simulink model "Nmpc_pathctl_casadi"  (R2022b)
settings: Solver=FixedStepAuto  StartTime=0.0  StopTime=25  FixedStep=.001  MaxStep=0.01  RelTol=1e-3
values from neighbouring files (symbols this model uses):
  xuanze = Input(15)    [NMPC_casadi_yhn.m]    (also in plotfig.m = 0)
libraries: Solver_SF x1
(part 1 of 11)
settings Model: SimulationMode=accelerator  Creator=Murad  LastModifiedBy=gfr_love_myf
settings SolverCC: AlgebraicLoopSolver=LineSearch
settings OptimizationCC: EfficientMapNaN2IntZero=off
settings DebuggingCC: UnconnectedInputMsg=warning  UnconnectedOutputMsg=warning  UnconnectedLineMsg=warning  SFMachineParentedDataDiag=warning
settings HardwareCC: TargetBitPerPointer=64  TargetBitPerSizeT=64  TargetBitPerPtrDiffT=64  TargetLongLongMode=on  TargetIntDivRoundTo=Zero  TargetEndianess=LittleEndian  TargetWordSize=64  TargetHWDeviceType=MATLAB Host  ProdEqTarget=off
settings ModelReferenceCC: EnableRefExpFcnMdlSchedulingChecks=on
settings SFSimCC: CustomCodeUndefinedFunction=UseInterfaceOnly
settings CodeAppCC: MaxIdLength=128
settings GRTTargetCC: TargetLangStandard=C89/C90 (ANSI)  CombineOutputUpdateFcns=off  GRTInterface=on

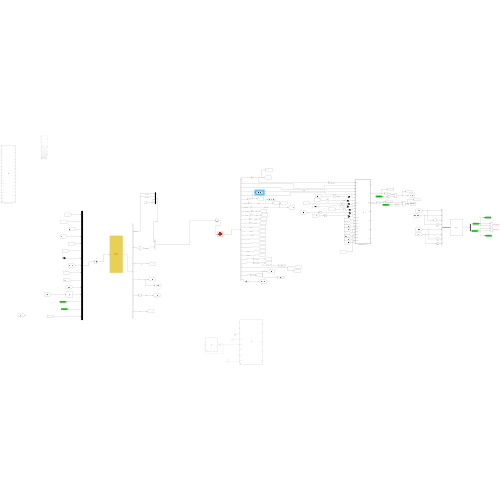
[thumbnail: Simulink's stored preview of the top-level diagram]
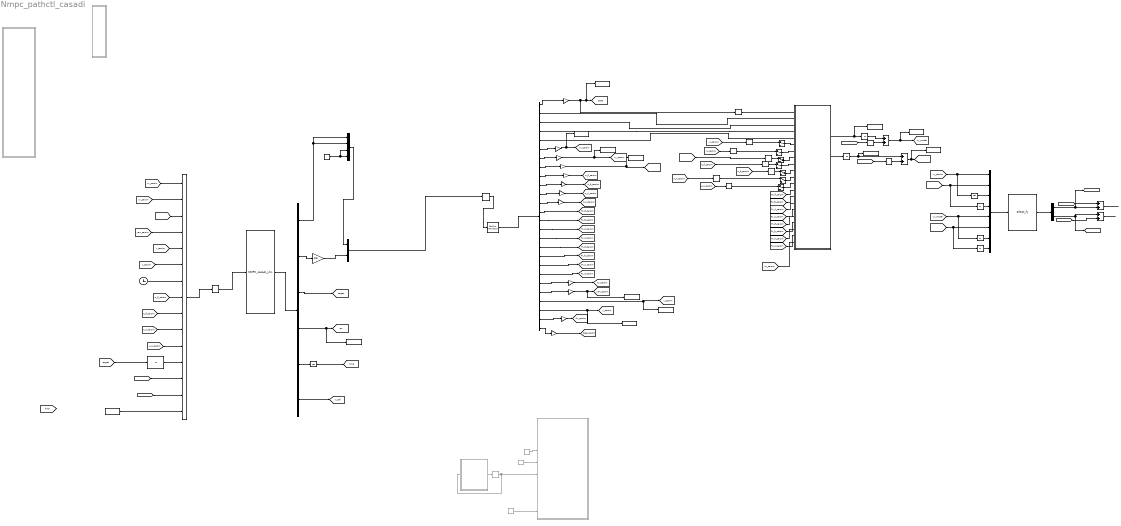
== system Nmpc_pathctl_casadi ==
  Add{1..4} (4 alike) : Sum
  Burckhardt轮胎侧向力_低附 : MATLAB Function  TreatAsAtomicUnit=on
  Burckhardt轮胎侧向力_低附1 : MATLAB Function  Commented=on  TreatAsAtomicUnit=on
  Bus Creator : BusCreator  Inputs=8
  CarSim S-Function : Solver_SF/CarSim S-Function  Priority=1  SIMFILE=simfile.sim  Run_RTs=off  vs_state_ind=Run  StopMode_ind=Vehicle Model
  Clock : Clock
  Constant : Constant  Value=0
  Constant1 : Constant  Commented=on  Value=10
  Constant2 : Constant  Commented=on  Value=10
  Constant3 : Constant  Commented=on  Value=10
  Constant4 : Constant  Value=xuanze
  Delay : Delay  Commented=on  DelayLength=1  InitialCondition=10
  Delay1 : Delay  DelayLength=1  InitialCondition=0
  Delay10 : Delay  DelayLength=15  InitialCondition=0
  Delay{2..5} (4 alike) : Delay  DelayLength=15  InitialCondition=8
  Delay6 : Delay  DelayLength=1  InitialCondition=10
  Delay7 : Delay  DelayLength=1  InitialCondition=0
  Delay8 : Delay  DelayLength=1  InitialCondition=0
  Delay9 : Delay  DelayLength=15  InitialCondition=0
  Demux : Demux  Outputs=2
  Demux1 : Demux  Outputs=6
  Demux2 : Demux  Outputs=26
  Gain : Gain  Gain=1/3.6
  Gain1 : Gain  Gain=1/3.6
  Gain10 : Gain  Gain=9.8
  Gain11 : Gain  Gain=400
  Gain{2,7,9,12} (4 alike) : Gain  Gain=pi/180
  Gain{3..6} (4 alike) : Gain  Gain=pi/30*0.3018
  Gain8 : Gain  Gain=9.8
  Interpreted MATLAB Function : MATLABFcn  MATLABFcn=NMPC_casadi_yhn  OutputDimensions=6  Output1D=off
  MATLAB Function1 : MATLAB Function  Commented=on  TreatAsAtomicUnit=on
  MATLAB Function2 : MATLAB Function  Commented=on  TreatAsAtomicUnit=on
  Manual Switch{,1..6} (7 alike) : ManualSwitch
  Mux : Mux  Inputs=2
  Mux1 : Mux  Inputs=15
  Mux2 : Mux
  Rate Transition1 : RateTransition  OutPortSampleTime=0.001
  Rate Transition2 : RateTransition  OutPortSampleTime=0.02
  S-Function1 : S-Function  FunctionName=adapt_fy  SFunctionDeploymentMode=off  EnableBusSupport=off
  To Workspace : ToWorkspace  VariableName=y_carsim  SaveFormat=Timeseries  SampleTime=-1
  To Workspace1 : ToWorkspace  VariableName=x_carsim  SaveFormat=Timeseries  SampleTime=-1
  To Workspace10 : ToWorkspace  VariableName=vy_data  SaveFormat=Timeseries  SampleTime=-1
  To Workspace11 : ToWorkspace  VariableName=vx_carsim  SaveFormat=Timeseries  SampleTime=-1
  To Workspace2 : ToWorkspace  VariableName=err  SaveFormat=Timeseries  SampleTime=-1
  To Workspace3 : ToWorkspace  VariableName=yaw  SaveFormat=Timeseries  SampleTime=-1
  To Workspace4 : ToWorkspace  VariableName=delta  SaveFormat=Timeseries  SampleTime=-1
  To Workspace5 : ToWorkspace  VariableName=vy_com  SaveFormat=Timeseries  SampleTime=-1
  To Workspace6 : ToWorkspace  VariableName=gamma_com  SaveFormat=Timeseries  SampleTime=-1
  To Workspace7 : ToWorkspace  VariableName=gamma_model  SaveFormat=Timeseries  SampleTime=-1
  To Workspace8 : ToWorkspace  VariableName=vy_model  SaveFormat=Timeseries  SampleTime=-1
  To Workspace9 : ToWorkspace  VariableName=gamma_data  SaveFormat=Timeseries  SampleTime=-1
  Unit Delay{1..6,12} (7 alike) : UnitDelay  SampleTime=-1  HasFrameUpgradeWarning=on
  Unit Delay11 : UnitDelay  InitialCondition=1  SampleTime=-1  HasFrameUpgradeWarning=on
  刘胜涛师兄路径跟踪 : Subsystem  Commented=on
  tag scope: Ax_carsim=global, Ay_carsim=global, Fx_fl_carsim=global, Fx_fr_carsim=global, Fx_rl_carsim=global, Fx_rr_carsim=global, Fy_fl_carsim=global, Fy_fr_carsim=global, Fy_rl_carsim=global, Fy_rr_carsim=global, beta_carsim=global, delta=global, err=global, gamma_carsim=global, gamma_com=global, gamma_model=global, target=global, time=global, vx_carsim=global, vy_carsim=global, vy_com=global, vy_model=global, w_fl_carsim=global, w_fr_carsim=global, w_ref=global, w_rl_carsim=global, w_rr_carsim=global, x_carsim=global, y_carsim=global, yaw_carsim=global
  wires:
  Burckhardt轮胎侧向力_低附/3(gamma) -> Unit Delay5/1  "gamma_model"
  CarSim S-Function/1 -> Demux2/1
  Demux2/1 -> Gain7/1  "delta_carsim"
  Demux2/2 -> Burckhardt轮胎侧向力_低附/2(Tc_fl)  "Tc_fl_carsim"
  Demux2/3 -> Burckhardt轮胎侧向力_低附/3(Tc_fr)  "Tc_fr_carsim"
  Demux2/4 -> Burckhardt轮胎侧向力_低附/4(Tc_rl)  "Tc_rl_carsim"
  Demux2/5 -> Burckhardt轮胎侧向力_低附/5(Tc_rr)  "Tc_rr_carsim"
  Demux2/6 -> Gain/1  "vx_carsim"
  Demux2/7 -> Gain1/1  "vy_carsim"
  Demux2/8 -> Gain2/1  "gamma_carsim"
  Demux2/9 -> Gain3/1  "w_fl_carsim"
  Demux2/10 -> Gain4/1  "w_fr_carsim"
  Demux2/11 -> Gain5/1  "w_rl_carsim"
  Demux2/12 -> Gain6/1  "w_rr_carsim"
  Gain1/1 -> To Workspace10/1, [vy_carsim]  "vy_carsim"
  Gain2/1 -> To Workspace9/1, [gamma_carsim]  "gamma_carsim"
  Gain3/1 -> [w_fl_carsim]  "w_fl_carsim"
  Gain4/1 -> [w_fr_carsim]  "w_fr_carsim"
  Gain5/1 -> [w_rl_carsim]  "w_rl_carsim"
  Gain6/1 -> [w_rr_carsim]  "w_rr_carsim"
  [vx_carsim] -> Delay6/1
  Manual Switch/1 -> Burckhardt轮胎侧向力_低附/6("vx ")
  Manual Switch1/1 -> Burckhardt轮胎侧向力_低附/7("vy ")
  [vy_carsim] -> Delay7/1
  [gamma_carsim] -> Delay8/1
  Manual Switch2/1 -> Burckhardt轮胎侧向力_低附/8("gamma ")
  Manual Switch3/1 -> Burckhardt轮胎侧向力_低附/9(w_fl)
  Manual Switch4/1 -> Burckhardt轮胎侧向力_低附/10(w_fr)
  Manual Switch5/1 -> Burckhardt轮胎侧向力_低附/11(w_rl)
  Manual Switch6/1 -> Burckhardt轮胎侧向力_低附/12(w_rr)
  Demux2/13 -> [Fy_fl_carsim]  "Fyfl_carsim"
  Demux2/14 -> [Fy_fr_carsim]  "Fyfr_carsim"
  Demux2/15 -> [Fy_rl_carsim]  "Fyrl_carsim"
  Demux2/16 -> [Fy_rr_carsim]  "Fyrr_carsim"
  Demux2/20 -> [Fx_rr_carsim]  "Fxrr_carsim"
  Demux2/18 -> [Fx_fr_carsim]  "Fxfr_carsim"
  Demux2/19 -> [Fx_rl_carsim]  "Fxrl_carsim"
  Demux2/17 -> [Fx_fl_carsim]  "Fxfl_carsim"
  [Fy_fl_carsim] -> Burckhardt轮胎侧向力_低附/13(fyfl_carsim)
  [Fy_fr_carsim] -> Burckhardt轮胎侧向力_低附/14(fyfr_carsim)
  [Fy_rl_carsim] -> Burckhardt轮胎侧向力_低附/15(fyrl_carsim)
  [Fy_rr_carsim] -> Burckhardt轮胎侧向力_低附/16(fyrr_carsim)
  [Fx_fl_carsim] -> Burckhardt轮胎侧向力_低附/17(fxfl_carsim)
  [Fx_fr_carsim] -> Burckhardt轮胎侧向力_低附/18(fxfr_carsim)
  [Fx_rl_carsim] -> Burckhardt轮胎侧向力_低附/19(fxrl_carsim)
  [Fx_rr_carsim] -> Burckhardt轮胎侧向力_低附/20(fxrr_carsim)
  Gain7/1 -> To Workspace4/1, [delta], Delay1/1  "delta_carsim"
  Demux2/21 -> Gain8/1  "Ay_carsim"
  Gain8/1 -> [Ay_carsim]  "Ay_carsim"
  [vy_carsim] -> Bus Creator/1, Unit Delay1/1
  [gamma_carsim] -> Unit Delay2/1, Bus Creator/2
  Unit Delay1/1 -> Bus Creator/3
  Unit Delay2/1 -> Bus Creator/4
  [vy_model] -> Unit Delay3/1, Bus Creator/5
  [gamma_model] -> Unit Delay4/1, Bus Creator/6
  Unit Delay4/1 -> Bus Creator/8
  Unit Delay3/1 -> Bus Creator/7
  Bus Creator/1 -> S-Function1/1
  Add2/1 -> ?  "Vy_com"
  S-Function1/1 -> Demux/1
  [vy_model] -> Add2/1
  Demux/2 -> [gamma_com], Add3/1
  Add3/1 -> ?  "gamma_com"
  Demux/1 -> Add2/2, [vy_com]
  [gamma_model] -> Add3/2
  Burckhardt轮胎侧向力_低附/2(vy) -> To Workspace8/1, Unit Delay6/1  "vy_model"
  [vy_com] -> Delay9/1
  Demux2/22 -> Gain9/1
  Gain9/1 -> To Workspace3/1, [yaw_carsim]  "yaw_carsim"
  Demux2/23 -> [x_carsim], To Workspace1/1  "x_carsim"
  Demux2/24 -> [y_carsim], To Workspace/1  "y_carsim"
  Demux2/25 -> Gain10/1
  Gain10/1 -> [Ax_carsim]  "Ax_carsim"
  Delay6/1 -> Manual Switch/1  "w_fl_model"
  Delay7/1 -> Manual Switch1/1  "w_fl_model"
  Delay8/1 -> Manual Switch2/1  "w_fl_model"
  [gamma_com] -> Delay10/1
  Add1/1 -> To Workspace5/1, [vy_model]  "Vy_com"
  Add4/1 -> To Workspace6/1, [gamma_model]  "gamma_com"
  [Ax_carsim] -> Burckhardt轮胎侧向力_低附/21(ax_carsim)
  [w_fl_carsim] -> Delay2/1
  [w_fr_carsim] -> Delay3/1
  [w_rl_carsim] -> Delay4/1
  [w_rr_carsim] -> Delay5/1
  Delay2/1 -> Manual Switch3/1
  Delay3/1 -> Manual Switch4/1
  Delay4/1 -> Manual Switch5/1
  Delay5/1 -> Manual Switch6/1
  Delay1/1 -> Burckhardt轮胎侧向力_低附/1(delta)  "w_fl_model"
  Delay9/1 -> Add1/2
  Delay10/1 -> Add4/2
  Interpreted MATLAB Function/1 -> Demux1/1
  Demux1/1 -> Mux2/2, Mux2/1  "delta_carsim"
  Constant/1 -> Mux2/3, Mux2/4
  Mux2/1 -> Mux/1
  Rate Transition1/1 -> CarSim S-Function/1
  Demux1/2 -> Gain11/1  "ax"
  Gain11/1 -> Mux/2  "T_emergine"
  [vx_carsim] -> Mux1/1
  [vy_carsim] -> Mux1/2
  [gamma_carsim] -> Mux1/3
  [yaw_carsim] -> Mux1/4
  [x_carsim] -> Mux1/5
  [y_carsim] -> Mux1/6
  Mux1/1 -> Rate Transition2/1
  Rate Transition2/1 -> Interpreted MATLAB Function/1
  [w_fl_carsim] -> Mux1/8
  [w_fr_carsim] -> Mux1/9
  [w_rl_carsim] -> Mux1/10
  [w_rr_carsim] -> Mux1/11
  Unit Delay5/1 -> To Workspace7/1, Add4/1  "w_fr_model"
  Unit Delay6/1 -> Add1/1  "w_fr_model"
  Clock/1 -> Mux1/7  "t"
  Demux1/3 -> [target]  "taget"
  Mux/1 -> Rate Transition1/1
  Unit Delay11/1 -> Mux1/12
  [target] -> Unit Delay11/1
  Demux1/4 -> To Workspace2/1, [err]  "err"
  Constant1/1 -> MATLAB Function1/8(target)
  MATLAB Function2/1(y) -> Delay/1
  Delay/1 -> MATLAB Function2/1(u), MATLAB Function1/5(curvepos0)  "x"
  Constant2/1 -> MATLAB Function1/4(lamada)
  Constant3/1 -> MATLAB Function1/3(z)
  Demux1/5 -> Unit Delay12/1
  Unit Delay12/1 -> [time]  "time"
  Demux2/26 -> Gain12/1
  Gain12/1 -> [beta_carsim]  "beta_carsim"
  Demux1/6 -> [w_ref]  "w_ref"
  Constant4/1 -> Mux1/15
  [vy_com] -> Mux1/13
  [gamma_com] -> Mux1/14
  Gain/1 -> To Workspace11/1, [vx_carsim]  "err"

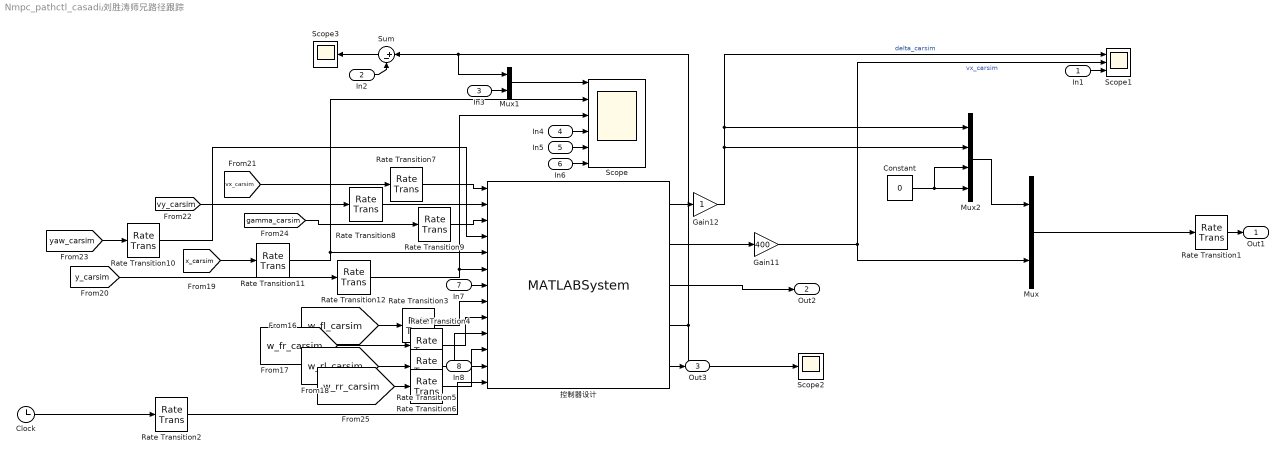
== system Nmpc_pathctl_casadi/刘胜涛师兄路径跟踪 ==
  In1 : Inport
  In2 : Inport  Port=2
  In3 : Inport  Port=3
  In4 : Inport  Port=4
  In5 : Inport  Port=5
  In6 : Inport  Port=6
  In7 : Inport  Port=7
  In8 : Inport  Port=8
  Clock : Clock
  Constant : Constant  Value=0
  Gain11 : Gain  Gain=400
  Gain12 : Gain
  Mux : Mux  Inputs=2
  Mux1 : Mux  Inputs=2
  Mux2 : Mux
  Rate Transition1 : RateTransition  OutPortSampleTime=0.001
  Rate Transition{2,7..11} (6 alike) : RateTransition  OutPortSampleTime=0.02
  Rate Transition{3..6,12} (5 alike) : RateTransition  OutPortSampleTime=0.1
  Scope : Scope  NumInputPorts=6
  Scope1 : Scope  NumInputPorts=3
  Scope2 : Scope
  Scope3 : Scope
  Sum : Sum  Inputs=|+-
  控制器设计 : MATLABSystem  System=NMPC_PCtl_casadi  SimulateUsing=Interpreted execution
      mask Type: NMPC_PCtl_casadi
      mask Display:
      | disp('NMPC_PCtl_casadi');
      | port_label('input',1,'xd_in');
      | port_label('input',2,'yd_in');
      | port_label('input',3,'yawd_in');
      | port_label('input',4,'yaw_in');
      | port_label('input',5,'x_in');
      | port_label('input',6,'y_in');
      | port_label('input',7,'w_fl');
      | port_label('input',8,'w_fr');
      | port_label('input',9,'w_rl');
      | port_label('input',10,'w_rr');
      | port_label('input',11,'vy_com');
      | port_label('input',12,'gamma_com');
      | port_label('input',13,'t');
      | port_label('output',1,'delta_out');
      | port_label('output',2,'acc_out');
      | port_label('output',3,'break_out');
      | port_label('output',4,'vref');
      | port_label('output',5,'target');
  Out1 : Outport
  Out2 : Outport  Port=2
  Out3 : Outport  Port=3
  wires:
  Mux/1 -> Rate Transition1/1
  In4/1 -> Scope/4
  Rate Transition1/1 -> Out1/1
  Mux2/1 -> Mux/1
  Gain12/1 -> Scope1/1, Mux2/1, Mux2/2  "delta_carsim"
  Rate Transition4/1 -> 控制器设计/9
  Clock/1 -> Rate Transition2/1
  Sum/1 -> Scope3/1
  控制器设计/1 -> Gain12/1
  Rate Transition12/1 -> 控制器设计/6, Scope/3
  [w_rl_carsim] -> Rate Transition5/1
  Mux1/1 -> Scope/1
  控制器设计/2 -> Gain11/1
  [gamma_carsim] -> Rate Transition9/1
  Gain11/1 -> Mux/2, Scope1/2  "vx_carsim"
  [yaw_carsim] -> Rate Transition10/1
  In1/1 -> Scope1/3
  控制器设计/4 -> Scope2/1, Mux1/1, Sum/1
  [vy_carsim] -> Rate Transition8/1
  Rate Transition9/1 -> 控制器设计/3
  Constant/1 -> Mux2/3, Mux2/4
  [x_carsim] -> Rate Transition11/1
  Rate Transition6/1 -> 控制器设计/11
  [w_fr_carsim] -> Rate Transition4/1
  控制器设计/3 -> Out2/1
  In8/1 -> 控制器设计/12
  [w_fl_carsim] -> Rate Transition3/1
  [y_carsim] -> Rate Transition12/1
  Rate Transition5/1 -> 控制器设计/10
  Rate Transition8/1 -> 控制器设计/2
  In5/1 -> Scope/5
  Rate Transition7/1 -> 控制器设计/1
  In3/1 -> Mux1/2
  [w_rr_carsim] -> Rate Transition6/1
  In6/1 -> Scope/6
  Rate Transition10/1 -> 控制器设计/4
  Rate Transition11/1 -> 控制器设计/5, Scope/2
  Rate Transition3/1 -> 控制器设计/8
  In2/1 -> Sum/2
  [vx_carsim] -> Rate Transition7/1
  Rate Transition2/1 -> 控制器设计/13
  In7/1 -> 控制器设计/7
  控制器设计/5 -> Out3/1
